simulink model "HareLynx"  (R2014b)
settings: Solver=ode45  StartTime=0.0  StopTime=80  MaxStep=0.1  RelTol=1e-3
libraries: simulink x1
settings Model: Creator=jeff  LastModifiedBy=jeff

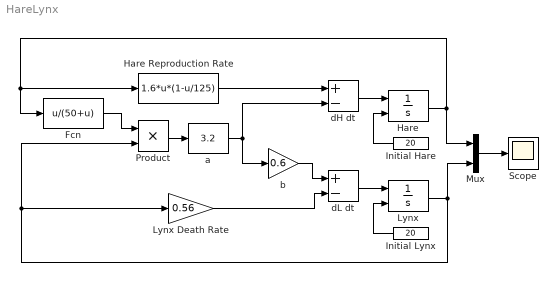
== system HareLynx ==
  Fcn : Fcn  Expr=u/(50+u)
  Hare : Integrator  InitialConditionSource=external  InitialCondition=20  LimitOutput=on  LowerSaturationLimit=0
  Hare Reproduction Rate : Fcn  Expr=1.6*u*(1-u/125)
  Initial Hare : Constant  Value=20
  Initial Lynx : Constant  Value=20
  Lynx : Integrator  InitialConditionSource=external  InitialCondition=20  LimitOutput=on  LowerSaturationLimit=0
  Lynx Death Rate : Gain  Gain=0.56
  Mux : Mux  Inputs=2
  Product : Product
  Scope : Scope
      settings: ShowLegends=on  TimeRange=80  YMin=0  YMax=90
  a : simulink/Math Operations/Slider Gain  low=0  gain=3.2  high=5
  "b " : Gain  Gain=0.6
  dH dt : Sum  Inputs=+-
  dL dt : Sum  Inputs=+-
  wires:
  dH dt/1 -> Hare/1
  dL dt/1 -> Lynx/1
  Lynx/1 -> Lynx Death Rate/1, Product/2, Mux/2
  Hare/1 -> Mux/1, Fcn/1, Hare Reproduction Rate/1
  Hare Reproduction Rate/1 -> dH dt/1
  Fcn/1 -> Product/1
  Product/1 -> a/1
  a/1 -> dH dt/2, "b "/1
  "b "/1 -> dL dt/1
  Lynx Death Rate/1 -> dL dt/2
  Mux/1 -> Scope/1
  Initial Hare/1 -> Hare/2
  Initial Lynx/1 -> Lynx/2
